simulink subsystem "PedalForce_to_Pressure"  (R2021b)
settings: Solver=VariableStepAuto  StartTime=0.0  StopTime=10.0  RelTol=1e-3
undefined symbols (not defined in the file): mPiston_Area_F, mPiston_Area_R, Pedal_Ratio
settings Model: Creator=tsuyoshi  LastModifiedBy=tsuyoshi

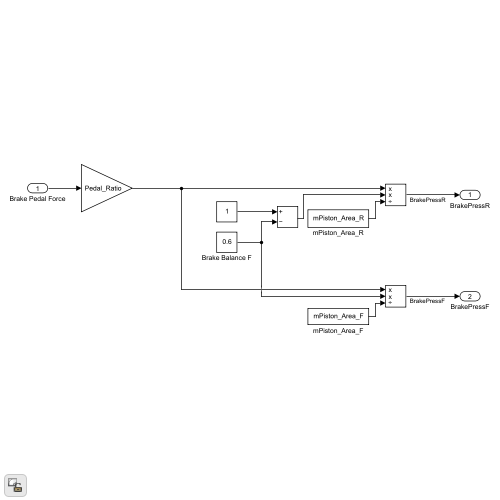
[thumbnail: Simulink's stored preview of the top-level diagram]
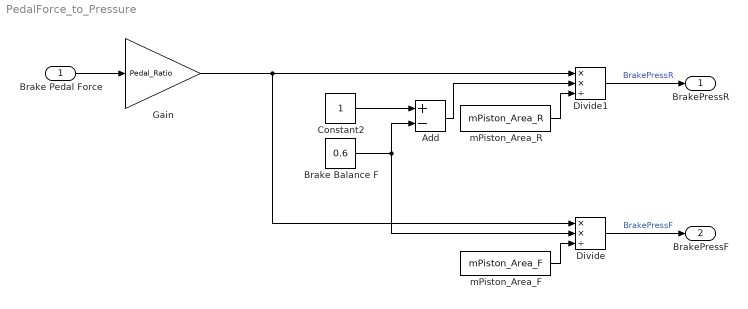
== system PedalForce_to_Pressure ==
  Brake Pedal Force : Inport
  Add : Sum  Inputs=+-
  Brake Balance F : Constant  Value=0.6
  Constant2 : Constant
  Divide : Product  Inputs=**/
  Divide1 : Product  Inputs=**/
  Gain : Gain  Gain=Pedal_Ratio
  mPiston_Area_F : Constant  Value=mPiston_Area_F
  mPiston_Area_R : Constant  Value=mPiston_Area_R
  BrakePressR : Outport
  BrakePressF : Outport  Port=2
  wires:
  mPiston_Area_F/1 -> Divide/3
  Divide1/1 -> BrakePressR/1  "BrakePressR"
  Gain/1 -> Divide/1, Divide1/1
  mPiston_Area_R/1 -> Divide1/3
  Brake Pedal Force/1 -> Gain/1
  Brake Balance F/1 -> Divide/2, Add/2
  Constant2/1 -> Add/1
  Add/1 -> Divide1/2
  Divide/1 -> BrakePressF/1  "BrakePressF"
